simulink model "ex11_model"  (R2021b)
settings: Solver=ode15s  StartTime=0.0  StopTime=1000.0  MaxStep=1  RelTol=1e-3  AbsTol=1e-3
values from neighbouring files (symbols this model uses):
  B = 1    [ex10.m]    (also in ex11.m = 6; ex4.m = [k0/T1 0 0]'; ex7.m = [k0/T1 0 0]')
  C = 1    [ex10.m]    (also in ex11.m = 0; ex7.m = [0 0 1])
  delta_fkul = 0    [ex10.m]    (also in ex11.m; ex8.m = 2; ex9.m = 2)
  fkul_0 = 35.7    [param.m]
  fp_0 = 35.7    [param.m]
  h1 = 8.3    [param.m]
  h2 = 21.0    (= 21)    [param.m]
  k0 = 1.0    (= 1)    [param.m]
  k1 = 2.0    (= 2)    [param.m]
  k2 = 1/30    (= 0.0333333333333)    [param.m]
  k3 = 0.4    [param.m]
  k4 = 1/300    (= 0.00333333333333)    [param.m]
  k5 = 0.6    [param.m]
  k6 = 0.6    [param.m]
  K_d = 20    [ex10.m]    (also in ex10_bode.m; ex11.m = 10; ex2.m = 0; ex3.m)
  K_dz = 0    [ex10.m]    (also in ex10_bode.m; ex11.m; ex8.m; ex9.m)
  K_i = 0.02    [ex10.m]    (also in ex10_bode.m; ex11.m; ex2.m = 0; ex3.m)
  k_in = 25.5    [ex10.m]    (also in ex11.m; param.m)
  K_iz = 0.02    [ex10.m]    (also in ex10_bode.m; ex11.m = 0.01; ex8.m = 0; ex9.m)
  k_out = 210    [ex10.m]    (also in ex11.m; param.m)
  K_p = 2    [ex10.m]    (also in ex10_bode.m; ex11.m; ex2.m = 0; ex3.m)
  K_pz = 0.3    [ex10.m]    (also in ex10_bode.m; ex11.m = 0.08; ex8.m = 0; ex9.m)
  ma_0 = 150000.0    (= 150000)    [param.m]
  omega_1 = 0.005    [ex10.m]    (also in ex11.m = 0.01)
  omega_2 = 0.2    [ex10.m]    (also in ex11.m)
  pa_0 = 10.0    (= 10)    [param.m]
  pcp = 13.0    (= 13)    [param.m]
  pk_0 = 91.0    (= 91)    [param.m]
  pkp_0 = 89.25    [param.m]
  pvp_0 = 3.0    (= 3)    [param.m]
  slope = 0    [ex10.m]    (also in ex11.m)
  T1 = 30.0    (= 30)    [param.m]
  Ts = 15.0    (= 15)    [param.m]
  z1_0 = 1    [ex10.m]    (also in ex11.m; ex4.m; ex7.m; ex8.m)
libraries: slpidlib x2, simulink x1
settings Model: Creator=meharju1  LastModifiedBy=tular
settings SolverCC: AutoScaleAbsTol=off  AlgebraicLoopSolver=TrustRegion
settings DataIOCC: SaveFormat=Array  SignalLoggingSaveFormat=ModelDataLogs  SaveOutput=off  TimeSaveName=t
settings OptimizationCC: DefaultParameterBehavior=Inlined  InlineInvariantSignals=on  ExpressionDepthLimit=2147483647  EfficientFloat2IntCast=on  LifeSpan=inf
settings DebuggingCC: SaveWithParameterizedLinksMsg=none  MultiTaskCondExecSysMsg=none  UniqueDataStoreMsg=error  StateNameClashWarn=warning  PregeneratedLibrarySubsystemCodeDiagnostic=none  StrictBusMsg=ErrorOnBusTreatedAsVector  SFUnexpectedBacktrackingDiag=warning  SFNoUnconditionalDefaultTransitionDiag=warning  SFExecutionAtInitializationDiag=none  SFMachineParentedDataDiag=warning  ArithmeticOperatorsInVariantConditions=warning
settings HardwareCC: ProdBitPerPointer=32  ProdBitPerSizeT=32  ProdBitPerPtrDiffT=32  ProdLargestAtomicFloat=None  ProdIntDivRoundTo=Undefined  ProdEndianess=Unspecified  ProdWordSize=32  ProdHWDeviceType=32-bit Generic  TargetUnknown=on
settings ModelReferenceCC: PropagateSignalLabelsOutOfModel=off
settings SFSimCC: SimUseLocalCustomCode=off  CustomCodeUndefinedFunction=UseInterfaceOnly
settings RTWCC: RTWUseLocalCustomCode=off
settings CodeAppCC: StateflowObjectComments=on
settings GRTTargetCC: TargetLangStandard=C89/C90 (ANSI)  CombineOutputUpdateFcns=off  GRTInterface=on
settings ConfigComp: CovMetricSettings=dw  CovSaveCumulativeToWorkspaceVar=on  CovSaveSingleToWorkspaceVar=on  CovExternalEMLEnable=off

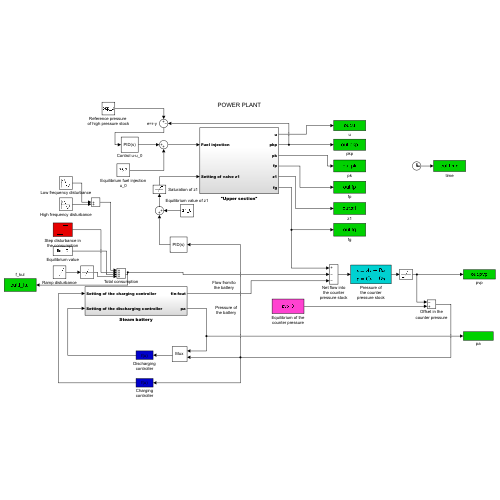
[thumbnail: Simulink's stored preview of the top-level diagram]
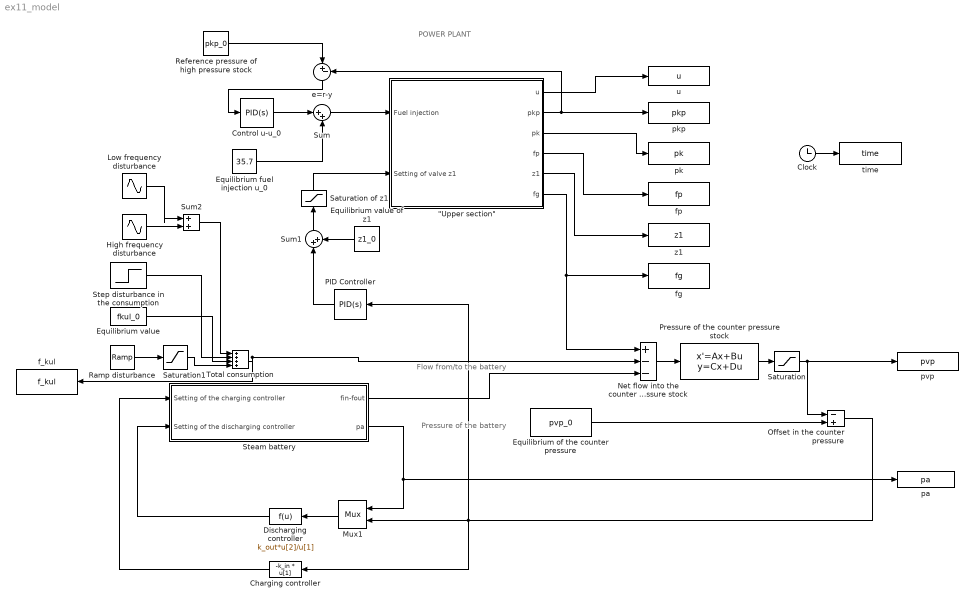
== system ex11_model ==
  note: POWER PLANT
  note: Flow from/to
      | the battery
  note: Pressure of
      | the battery
  "\"Upper section\"" : Subsystem
  Charging controller : Fcn  Expr=-k_in * u[1]
  Clock : Clock
  Control u-u_0 : slpidlib/PID Controller  Controller=PID  Form=Parallel  TimeDomain=Continuous-time  UseExternalTs=off  SampleTime=-1  IntegratorMethod=Forward Euler  FilterMethod=Forward Euler  ControllerParametersSource=internal  P=K_p  I=K_i  D=K_d  UseFilter=on  N=100  TunerSelectOption=Transfer Function Based (PID Tuner App)  InitialConditionSource=internal  InitialConditionForIntegrator=0  InitialConditionForFilter=0  DifferentiatorICPrevScaledInput=0  ExternalReset=none  TrackingMode=off  Kt=1  LimitOutput=off  SatLimitsSource=internal  UpperSaturationLimit=inf  LowerSaturationLimit=-inf  LinearizeAsGain=on  AntiWindupMode=none  Kb=1  POutMin=[]  POutMax=[]  IOutMin=[]  IOutMax=[]  DOutMin=[]  DOutMax=[]  NOutMin=[]  NOutMax=[]  SumOutMin=[]  SumOutMax=[]  SaturationOutMin=[]  SaturationOutMax=[]  PParamMin=[]  PParamMax=[]  IParamMin=[]  IParamMax=[]  DParamMin=[]  DParamMax=[]  NParamMin=[]  NParamMax=[]  KbParamMin=[]  KbParamMax=[]  KtParamMin=[]  KtParamMax=[]  KbOutMin=[]  KbOutMax=[]  KtOutMin=[]  KtOutMax=[]  IntegratorOutMin=[]  IntegratorOutMax=[]  FilterOutMin=[]  FilterOutMax=[]  SumI1OutMin=[]  SumI1OutMax=[]  SumI2OutMin=[]  SumI2OutMax=[]  SumI3OutMin=[]  SumI3OutMax=[]  SumI4OutMin=[]  SumI4OutMax=[]  SumDOutMin=[]  SumDOutMax=[]  DifferentiatorOutMin=[]  DifferentiatorOutMax=[]  FilterDiffOutCoefMin=[]  FilterDiffOutCoefMax=[]  ReciprocalOutMin=[]  ReciprocalOutMax=[]  SumDenOutMin=[]  SumDenOutMax=[]  SumNumOutMin=[]  SumNumOutMax=[]  DivideOutMin=[]  DivideOutMax=[]  UdiffTsProdOutMin=[]  UdiffTsProdOutMax=[]  NTsProdOutMin=[]  NTsProdOutMax=[]  UintegralTsProdOutMin=[]  UintegralTsProdOutMax=[]  UngainTsProdOutMin=[]  UngainTsProdOutMax=[]  IntegratorContinuousStateAttributes=''  IntegratorStateMustResolveToSignalObject=off  IntegratorRTWStateStorageClass=Auto  FilterContinuousStateAttributes=''  FilterStateMustResolveToSignalObject=off  FilterRTWStateStorageClass=Auto  ParallelPVariant=InternalParameters  IdealPVariant=Disabled  IVariant=InternalParameters  DVariant=InternalParameters  IntegratorVariant=Continuous  SatVariant=Disabled  AWVariant=Passthrough  PCopyVariant=Disabled  TRVariant=Disabled  FdbkBlocksVariant=Forward  IdealPFdbkVariant=Disabled  SatFdbkVariant=Disabled  DerivativeFilterVariant=ContFilter  NVariant=InternalParameters  NCopyVariant=Disabled  FilterICVariant=InternalICsFilter  IntegratorICVariant=InternalICs  ExternalResetVariant=Disabled  TRSumVariant=Passthrough  SumFdbkVariant=Disabled  SumVariant=Sum_PID  TsampFilterVariant=InternalTs  TsampNgainVariant=Passthrough  TsampIntegralVariant=Passthrough  ExternalSaturationOutDataTypeStr=Inherit: Same as second input
  Discharging controller : Fcn  Expr=k_out*u[2]/u[1]
  Equilibrium fuel injection u_0 : Constant  Value=35.7
  Equilibrium of the counter pressure : Constant  Value=pvp_0
  Equilibrium value : Constant  Value=fkul_0
  Equilibrium value of z1 : Constant  Value=z1_0
  High frequency disturbance : Sin  Amplitude=C  Frequency=omega_2  SampleTime=0
  Low frequency disturbance : Sin  Amplitude=B  Frequency=omega_1  SampleTime=0
  Mux1 : Mux  Inputs=2
  Net flow into the counter pressure stock : Sum  Inputs=+--  InputSameDT=on  SaturateOnIntegerOverflow=on  OutDataTypeStr=Inherit: Same as first input
  Offset in the counter pressure : Sum  Inputs=-+  InputSameDT=on  SaturateOnIntegerOverflow=on  OutDataTypeStr=Inherit: Same as first input
  PID Controller : slpidlib/PID Controller  Controller=PID  Form=Parallel  TimeDomain=Continuous-time  UseExternalTs=off  SampleTime=-1  IntegratorMethod=Forward Euler  FilterMethod=Forward Euler  ControllerParametersSource=internal  P=K_pz  I=K_iz  D=K_dz  UseFilter=on  N=100  TunerSelectOption=Transfer Function Based (PID Tuner App)  InitialConditionSource=internal  InitialConditionForIntegrator=0  InitialConditionForFilter=0  DifferentiatorICPrevScaledInput=0  ExternalReset=none  TrackingMode=off  Kt=1  LimitOutput=off  SatLimitsSource=internal  UpperSaturationLimit=inf  LowerSaturationLimit=-inf  LinearizeAsGain=on  AntiWindupMode=none  Kb=1  POutMin=[]  POutMax=[]  IOutMin=[]  IOutMax=[]  DOutMin=[]  DOutMax=[]  NOutMin=[]  NOutMax=[]  SumOutMin=[]  SumOutMax=[]  SaturationOutMin=[]  SaturationOutMax=[]  PParamMin=[]  PParamMax=[]  IParamMin=[]  IParamMax=[]  DParamMin=[]  DParamMax=[]  NParamMin=[]  NParamMax=[]  KbParamMin=[]  KbParamMax=[]  KtParamMin=[]  KtParamMax=[]  KbOutMin=[]  KbOutMax=[]  KtOutMin=[]  KtOutMax=[]  IntegratorOutMin=[]  IntegratorOutMax=[]  FilterOutMin=[]  FilterOutMax=[]  SumI1OutMin=[]  SumI1OutMax=[]  SumI2OutMin=[]  SumI2OutMax=[]  SumI3OutMin=[]  SumI3OutMax=[]  SumI4OutMin=[]  SumI4OutMax=[]  SumDOutMin=[]  SumDOutMax=[]  DifferentiatorOutMin=[]  DifferentiatorOutMax=[]  FilterDiffOutCoefMin=[]  FilterDiffOutCoefMax=[]  ReciprocalOutMin=[]  ReciprocalOutMax=[]  SumDenOutMin=[]  SumDenOutMax=[]  SumNumOutMin=[]  SumNumOutMax=[]  DivideOutMin=[]  DivideOutMax=[]  UdiffTsProdOutMin=[]  UdiffTsProdOutMax=[]  NTsProdOutMin=[]  NTsProdOutMax=[]  UintegralTsProdOutMin=[]  UintegralTsProdOutMax=[]  UngainTsProdOutMin=[]  UngainTsProdOutMax=[]  IntegratorContinuousStateAttributes=''  IntegratorStateMustResolveToSignalObject=off  IntegratorRTWStateStorageClass=Auto  FilterContinuousStateAttributes=''  FilterStateMustResolveToSignalObject=off  FilterRTWStateStorageClass=Auto  ParallelPVariant=InternalParameters  IdealPVariant=Disabled  IVariant=InternalParameters  DVariant=InternalParameters  IntegratorVariant=Continuous  SatVariant=Disabled  AWVariant=Passthrough  PCopyVariant=Disabled  TRVariant=Disabled  FdbkBlocksVariant=Forward  IdealPFdbkVariant=Disabled  SatFdbkVariant=Disabled  DerivativeFilterVariant=ContFilter  NVariant=InternalParameters  NCopyVariant=Disabled  FilterICVariant=InternalICsFilter  IntegratorICVariant=InternalICs  ExternalResetVariant=Disabled  TRSumVariant=Passthrough  SumFdbkVariant=Disabled  SumVariant=Sum_PID  TsampFilterVariant=InternalTs  TsampNgainVariant=Passthrough  TsampIntegralVariant=Passthrough  ExternalSaturationOutDataTypeStr=Inherit: Same as second input
  Pressure of the counter pressure stock : StateSpace  A=0  B=k4  D=0  InitialCondition=pvp_0
  Ramp disturbance : simulink/Sources/Ramp  slope=slope  start=200  InitialOutput=0
  Reference pressure of high pressure stock : Constant  Value=pkp_0
  Saturation : Saturate  UpperLimit=100000  LowerLimit=0
  Saturation of z1 : Saturate  UpperLimit=1.2  LowerLimit=0.8
  Saturation1 : Saturate  UpperLimit=7  LowerLimit=-7
  Steam battery : Subsystem
  Step disturbance in the consumption : Step  Time=200  After=delta_fkul  SampleTime=0
  Sum : Sum  Inputs=|++
  Sum1 : Sum  Inputs=|++
  Sum2 : Sum  Inputs=|++
  Total consumption : Sum  Inputs=++++  InputSameDT=on  SaturateOnIntegerOverflow=on  OutDataTypeStr=Inherit: Same as first input
  e=r-y : Sum  Inputs=|+-
  f_kul : ToWorkspace  VariableName=f_kul
      settings: MaxDataPoints=2000
  fg : ToWorkspace  VariableName=fg
      settings: MaxDataPoints=2000
  fp : ToWorkspace  VariableName=fp
      settings: MaxDataPoints=2000
  pa : ToWorkspace  VariableName=pa
      settings: MaxDataPoints=2000
  pk : ToWorkspace  VariableName=pk
      settings: MaxDataPoints=2000
  pkp : ToWorkspace  VariableName=pkp
      settings: MaxDataPoints=2000
  pvp : ToWorkspace  VariableName=pvp
      settings: MaxDataPoints=2000
  time : ToWorkspace  VariableName=time
      settings: MaxDataPoints=2000
  u : ToWorkspace  VariableName=u
      settings: MaxDataPoints=2000
  z1 : ToWorkspace  VariableName=z1
      settings: MaxDataPoints=2000
  wires:
  Net flow into the counter pressure stock/1 -> Pressure of the counter pressure stock/1
  Mux1/1 -> Discharging controller/1
  Equilibrium of the counter pressure/1 -> Offset in the counter pressure/2
  Steam battery/2(pa) -> pa/1, Mux1/1
  Total consumption/1 -> f_kul/1, Net flow into the counter pressure stock/2
  Steam battery/1(fin-fout) -> Net flow into the counter pressure stock/3
  Discharging controller/1 -> Steam battery/2(Setting of the discharging controller)
  Offset in the counter pressure/1 -> PID Controller/1, Mux1/2, Charging controller/1
  "\"Upper section\""/1(u) -> u/1
  "\"Upper section\""/2(pkp) -> pkp/1, e=r-y/2
  "\"Upper section\""/3(pk) -> pk/1
  "\"Upper section\""/4(fp) -> fp/1
  Equilibrium fuel injection u_0/1 -> Sum/2
  Pressure of the counter pressure stock/1 -> Saturation/1
  Saturation/1 -> pvp/1, Offset in the counter pressure/1
  "\"Upper section\""/6(fg) -> Net flow into the counter pressure stock/1, fg/1
  "\"Upper section\""/5(z1) -> z1/1
  Charging controller/1 -> Steam battery/1(Setting of the charging controller)
  Clock/1 -> time/1
  Reference pressure of high pressure stock/1 -> e=r-y/1
  Control u-u_0/1 -> Sum/1
  Sum/1 -> "\"Upper section\""/1(Fuel injection)
  Saturation of z1/1 -> "\"Upper section\""/2(Setting of valve z1)
  Sum1/1 -> Saturation of z1/1
  Equilibrium value of z1/1 -> Sum1/2
  PID Controller/1 -> Sum1/1
  Equilibrium value/1 -> Total consumption/3
  Step disturbance in the consumption/1 -> Total consumption/2
  e=r-y/1 -> Control u-u_0/1
  High frequency disturbance/1 -> Sum2/2
  Low frequency disturbance/1 -> Sum2/1
  Sum2/1 -> Total consumption/1
  Ramp disturbance/1 -> Saturation1/1
  Saturation1/1 -> Total consumption/4

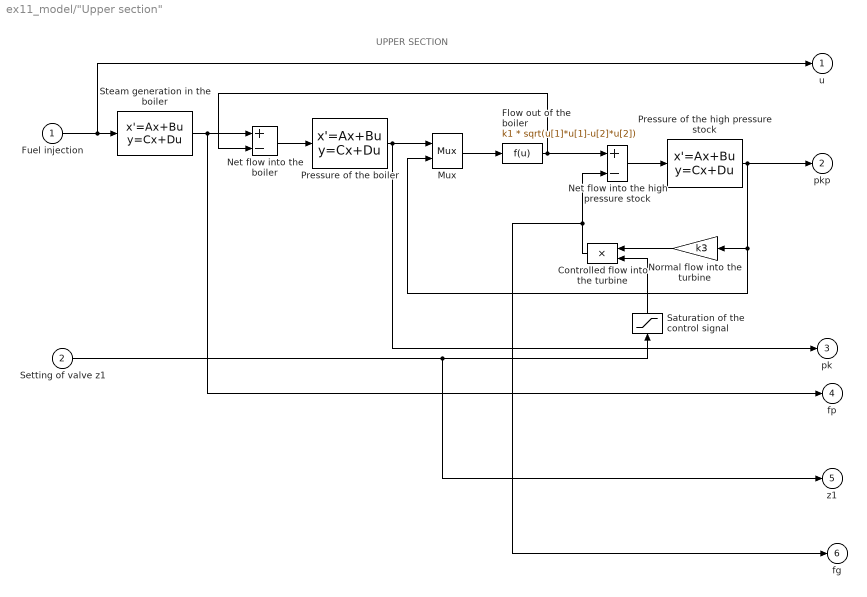
== system ex11_model/"Upper section" ==
  note: UPPER SECTION
  Fuel injection : Inport
  Setting of valve z1 : Inport  Port=2
  Controlled flow into the turbine : Product  InputSameDT=on  RndMeth=Zero  SaturateOnIntegerOverflow=on  OutDataTypeStr=Inherit: Same as first input
  Flow out of the boiler : Fcn  Expr=k1 * sqrt(u[1]*u[1]-u[2]*u[2])
  Mux : Mux  Inputs=2
  Net flow into the boiler : Sum  Inputs=+-  InputSameDT=on  SaturateOnIntegerOverflow=on  OutDataTypeStr=Inherit: Same as first input
  Net flow into the high pressure stock : Sum  Inputs=+-  InputSameDT=on  SaturateOnIntegerOverflow=on  OutDataTypeStr=Inherit: Same as first input
  Normal flow into the turbine : Gain  Gain=k3  SaturateOnIntegerOverflow=on  OutDataTypeStr=Inherit: Same as input  ParamDataTypeStr=Inherit: Same as input
  Pressure of the boiler : StateSpace  A=0  B=1/Ts  D=0  InitialCondition=pk_0
  Pressure of the high pressure stock : StateSpace  A=0  B=k2  D=0  InitialCondition=pkp_0
  Saturation of the control signal : Saturate  UpperLimit=1.2  LowerLimit=0.8
  Steam generation in the boiler : StateSpace  A=-1/T1  B=k0 / T1  D=0  InitialCondition=fp_0
  u : Outport  VectorParamsAs1DForOutWhenUnconnected=off
  pkp : Outport  Port=2  VectorParamsAs1DForOutWhenUnconnected=off
  pk : Outport  Port=3  VectorParamsAs1DForOutWhenUnconnected=off
  fp : Outport  Port=4  VectorParamsAs1DForOutWhenUnconnected=off
  z1 : Outport  Port=5  VectorParamsAs1DForOutWhenUnconnected=off
  fg : Outport  Port=6  VectorParamsAs1DForOutWhenUnconnected=off
  wires:
  Saturation of the control signal/1 -> Controlled flow into the turbine/2
  Normal flow into the turbine/1 -> Controlled flow into the turbine/1
  Pressure of the high pressure stock/1 -> Normal flow into the turbine/1, Mux/2, pkp/1
  Net flow into the high pressure stock/1 -> Pressure of the high pressure stock/1
  Flow out of the boiler/1 -> Net flow into the boiler/2, Net flow into the high pressure stock/1
  Mux/1 -> Flow out of the boiler/1
  Net flow into the boiler/1 -> Pressure of the boiler/1
  Pressure of the boiler/1 -> Mux/1, pk/1
  Steam generation in the boiler/1 -> Net flow into the boiler/1, fp/1
  Controlled flow into the turbine/1 -> Net flow into the high pressure stock/2, fg/1
  Fuel injection/1 -> Steam generation in the boiler/1, u/1
  Setting of valve z1/1 -> Saturation of the control signal/1, z1/1

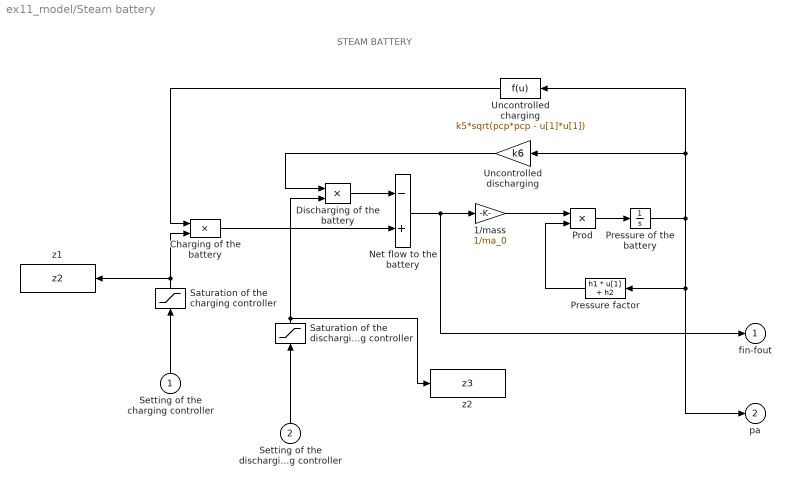
== system ex11_model/Steam battery ==
  note: STEAM BATTERY
  Setting of the charging controller : Inport
  Setting of the discharging controller : Inport  Port=2
  1/mass : Gain  Gain=1/ma_0  SaturateOnIntegerOverflow=on  OutDataTypeStr=Inherit: Same as input  ParamDataTypeStr=Inherit: Same as input
  Charging of the battery : Product  InputSameDT=on  RndMeth=Zero  SaturateOnIntegerOverflow=on  OutDataTypeStr=Inherit: Same as first input
  Discharging of the battery : Product  InputSameDT=on  RndMeth=Zero  SaturateOnIntegerOverflow=on  OutDataTypeStr=Inherit: Same as first input
  Net flow to the battery : Sum  Inputs=-+  InputSameDT=on  SaturateOnIntegerOverflow=on  OutDataTypeStr=Inherit: Same as first input
  Pressure factor : Fcn  Expr="h1 * u[1]  + h2"
  Pressure of the battery : Integrator  InitialCondition=pa_0
  Prod : Product  InputSameDT=on  RndMeth=Zero  SaturateOnIntegerOverflow=on  OutDataTypeStr=Inherit: Same as first input
  Saturation of the charging controller : Saturate  UpperLimit=1  LowerLimit=0
  Saturation of the discharging controller : Saturate  UpperLimit=1  LowerLimit=0
  Uncontrolled charging : Fcn  Expr=k5*sqrt(pcp*pcp - u[1]*u[1])
  Uncontrolled discharging : Gain  Gain=k6  SaturateOnIntegerOverflow=on  OutDataTypeStr=Inherit: Same as input  ParamDataTypeStr=Inherit: Same as input
  z1 : ToWorkspace  VariableName=z2
      settings: MaxDataPoints=2000
  z2 : ToWorkspace  VariableName=z3
      settings: MaxDataPoints=2000
  fin-fout : Outport  VectorParamsAs1DForOutWhenUnconnected=off
  pa : Outport  Port=2  VectorParamsAs1DForOutWhenUnconnected=off
  wires:
  Saturation of the charging controller/1 -> z1/1, Charging of the battery/2
  Saturation of the discharging controller/1 -> z2/1, Discharging of the battery/2
  Uncontrolled discharging/1 -> Discharging of the battery/1
  Charging of the battery/1 -> Net flow to the battery/2
  Uncontrolled charging/1 -> Charging of the battery/1
  1/mass/1 -> Prod/1
  Pressure factor/1 -> Prod/2
  Prod/1 -> Pressure of the battery/1
  Pressure of the battery/1 -> Pressure factor/1, pa/1, Uncontrolled charging/1, Uncontrolled discharging/1
  Setting of the discharging controller/1 -> Saturation of the discharging controller/1
  Setting of the charging controller/1 -> Saturation of the charging controller/1
  Net flow to the battery/1 -> fin-fout/1, 1/mass/1
  Discharging of the battery/1 -> Net flow to the battery/1
